simulink model "SecRwLtStBkReclnHolderChk"  (R2018b)
settings: Solver=FixedStepDiscrete  StartTime=0.0  StopTime=10.0  FixedStep=0.01  RelTol=1e-3
libraries: simulink x2
settings Model: Creator=sn2xws  LastModifiedBy=sn2xws
settings Model: ModifiedHistory=|
  | 2023/11/7
  | bug 555794 童锁需要停止21-26
  | 2024.5.8 V3.0.0 557 eze模式变更
  | 2024.9.9 V3.0.1 新增Md56
  | 25.7.7 V3.13.0 新增Md61 Md62
settings DataIOCC: SaveFormat=StructureWithTime
settings OptimizationCC: DefaultParameterBehavior=Inlined  EnhancedBackFolding=on  PassReuseOutputArgsAs=Individual arguments  ZeroExternalMemoryAtStartup=off  ZeroInternalMemoryAtStartup=off  OptimizeBlockOrder=speed  DifferentSizesBufferReuse=on  OptimizationCustomize=off
settings DebuggingCC: ParameterTunabilityLossMsg=error
settings ModelReferenceCC: ModelReferenceNumInstancesAllowed=Single
settings SFSimCC: MATLABDynamicMemAlloc=off
settings RTWCC: SystemTargetFile=autosar.tlc  GenCodeOnly=on  TemplateMakefile=ert_default_tmf  Description=AUTOSAR  GenerateReport=on  IncludeHyperlinkInReport=on  LaunchReport=on  GenerateTraceInfo=on  GenerateTraceReport=on  GenerateTraceReportSl=on  GenerateTraceReportSf=on  GenerateTraceReportEml=on  GenerateCodeMetricsReport=on
settings CodeAppCC: ForceParamTrailComments=on  IgnoreCustomStorageClasses=off  OperatorAnnotations=on  SimulinkDataObjDesc=on  SFDataObjDesc=on  InsertBlockDesc=on
settings STFCustomTargetCC: TargetLangStandard=C99 (ISO)  MultiwordLength=256  ParMdlRefBuildCompliant=on  CompOptLevelCompliant=on  IncludeMdlTerminateFcn=off  CombineOutputUpdateFcns=on  SuppressErrorStatus=on  ERTCustomFileBanners=on  SupportNonFinite=off  SupportComplex=off  SupportContinuousTime=off  SupportNonInlinedSFcns=off  RemoveResetFunc=on  MATLABClassNameForMDSCustomization=Simulink.SoftwareTarget.ERTCustomization  AutosarCompliant=on  UseToolchainInfoCompliant=on  LookupTableObjectStructAxisOrder=2,1,3,4,...  LUTObjectStructOrderEvenSpacing=Size,Table,Breakpoints  SystemTargetFile=autosar.tlc
settings ERTTargetCC: TargetLangStandard=C99 (ISO)  ConcurrentExecutionCompliant=off  IncludeMdlTerminateFcn=off  SuppressErrorStatus=on  SupportNonFinite=off  SupportComplex=off  ModelStepFunctionPrototypeControlCompliant=off  CPPClassGenCompliant=off  AutosarCompliant=on  LookupTableObjectStructAxisOrder=2,1,3,4,...  LUTObjectStructOrderEvenSpacing=Size,Table,Breakpoints  InlinedParameterPlacement=NonHierarchical  ERTCustomFileTemplate=example_file_process.tlc  ERTFilePackagingFormat=Compact

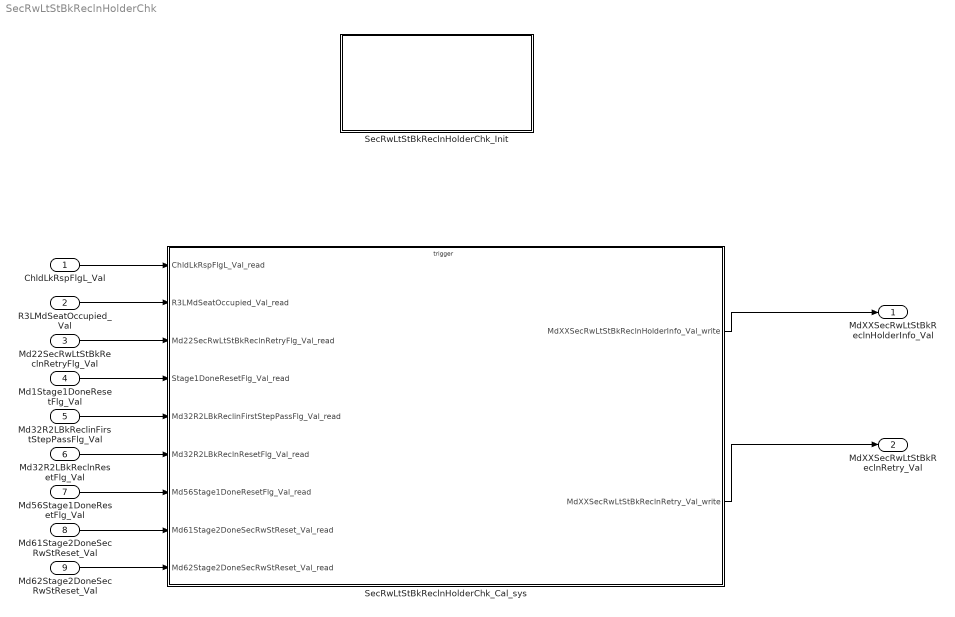
== system SecRwLtStBkReclnHolderChk ==
  ChldLkRspFlgL_Val : Inport  OutDataTypeStr=boolean  PortDimensions=1
  R3LMdSeatOccupied_Val : Inport  Port=2  OutDataTypeStr=boolean  PortDimensions=1
  Md22SecRwLtStBkReclnRetryFlg_Val : Inport  Port=3  OutDataTypeStr=boolean  PortDimensions=1
  Md1Stage1DoneResetFlg_Val : Inport  Port=4  OutDataTypeStr=boolean  PortDimensions=1
  Md32R2LBkReclinFirstStepPassFlg_Val : Inport  Port=5  OutDataTypeStr=boolean  PortDimensions=1
  Md32R2LBkReclnResetFlg_Val : Inport  Port=6  OutDataTypeStr=boolean  PortDimensions=1
  Md56Stage1DoneResetFlg_Val : Inport  Port=7  OutDataTypeStr=boolean  PortDimensions=1
  Md61Stage2DoneSecRwStReset_Val : Inport  Port=8  OutDataTypeStr=boolean  PortDimensions=1
  Md62Stage2DoneSecRwStReset_Val : Inport  Port=9  OutDataTypeStr=boolean  PortDimensions=1
  SecRwLtStBkReclnHolderChk_Cal_sys : Subsystem
  SecRwLtStBkReclnHolderChk_Init : Subsystem
  MdXXSecRwLtStBkReclnHolderInfo_Val : Outport  OutDataTypeStr=uint32  PortDimensions=1
  MdXXSecRwLtStBkReclnRetry_Val : Outport  Port=2  OutDataTypeStr=uint32  PortDimensions=1
  wires:
  ChldLkRspFlgL_Val/1 -> SecRwLtStBkReclnHolderChk_Cal_sys/1(ChldLkRspFlgL_Val_read)
  R3LMdSeatOccupied_Val/1 -> SecRwLtStBkReclnHolderChk_Cal_sys/2(R3LMdSeatOccupied_Val_read)
  SecRwLtStBkReclnHolderChk_Cal_sys/1(MdXXSecRwLtStBkReclnHolderInfo_Val_write) -> MdXXSecRwLtStBkReclnHolderInfo_Val/1
  Md22SecRwLtStBkReclnRetryFlg_Val/1 -> SecRwLtStBkReclnHolderChk_Cal_sys/3(Md22SecRwLtStBkReclnRetryFlg_Val_read)
  SecRwLtStBkReclnHolderChk_Cal_sys/2(MdXXSecRwLtStBkReclnRetry_Val_write) -> MdXXSecRwLtStBkReclnRetry_Val/1
  Md1Stage1DoneResetFlg_Val/1 -> SecRwLtStBkReclnHolderChk_Cal_sys/4(Stage1DoneResetFlg_Val_read)
  Md32R2LBkReclinFirstStepPassFlg_Val/1 -> SecRwLtStBkReclnHolderChk_Cal_sys/5(Md32R2LBkReclinFirstStepPassFlg_Val_read)
  Md32R2LBkReclnResetFlg_Val/1 -> SecRwLtStBkReclnHolderChk_Cal_sys/6(Md32R2LBkReclnResetFlg_Val_read)
  Md56Stage1DoneResetFlg_Val/1 -> SecRwLtStBkReclnHolderChk_Cal_sys/7(Md56Stage1DoneResetFlg_Val_read)
  Md61Stage2DoneSecRwStReset_Val/1 -> SecRwLtStBkReclnHolderChk_Cal_sys/8(Md61Stage2DoneSecRwStReset_Val_read)
  Md62Stage2DoneSecRwStReset_Val/1 -> SecRwLtStBkReclnHolderChk_Cal_sys/9(Md62Stage2DoneSecRwStReset_Val_read)

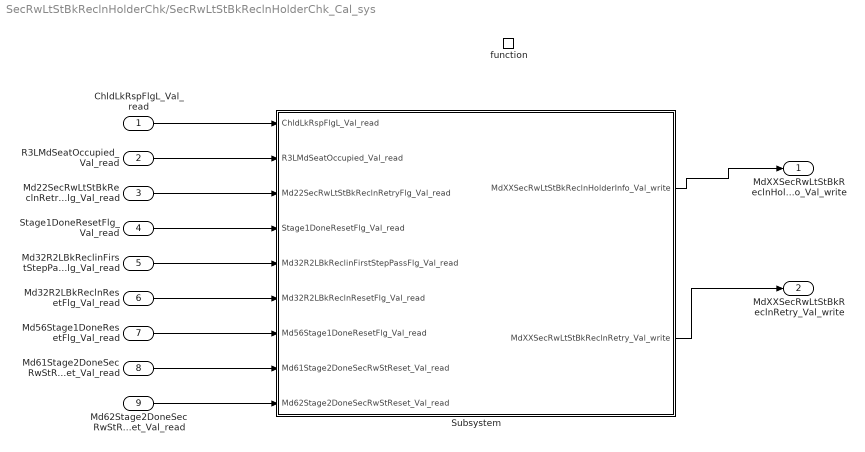
== system SecRwLtStBkReclnHolderChk/SecRwLtStBkReclnHolderChk_Cal_sys ==
  ChldLkRspFlgL_Val_read : Inport
  R3LMdSeatOccupied_Val_read : Inport  Port=2
  Md22SecRwLtStBkReclnRetryFlg_Val_read : Inport  Port=3
  Stage1DoneResetFlg_Val_read : Inport  Port=4
  Md32R2LBkReclinFirstStepPassFlg_Val_read : Inport  Port=5
  Md32R2LBkReclnResetFlg_Val_read : Inport  Port=6
  Md56Stage1DoneResetFlg_Val_read : Inport  Port=7
  Md61Stage2DoneSecRwStReset_Val_read : Inport  Port=8
  Md62Stage2DoneSecRwStReset_Val_read : Inport  Port=9
  function : TriggerPort  TriggerType=function-call  IsSimulinkFunction=on  FunctionName=SecRwLtStBkReclnHolderChk_Cal  VariantControl=(inherit)
  Subsystem : Subsystem
  MdXXSecRwLtStBkReclnHolderInfo_Val_write : Outport
      settings: EnsureOutportIsVirtual=on
  MdXXSecRwLtStBkReclnRetry_Val_write : Outport  Port=2
      settings: EnsureOutportIsVirtual=on
  wires:
  Subsystem/1(MdXXSecRwLtStBkReclnHolderInfo_Val_write) -> MdXXSecRwLtStBkReclnHolderInfo_Val_write/1
  ChldLkRspFlgL_Val_read/1 -> Subsystem/1(ChldLkRspFlgL_Val_read)
  R3LMdSeatOccupied_Val_read/1 -> Subsystem/2(R3LMdSeatOccupied_Val_read)
  Md22SecRwLtStBkReclnRetryFlg_Val_read/1 -> Subsystem/3(Md22SecRwLtStBkReclnRetryFlg_Val_read)
  Subsystem/2(MdXXSecRwLtStBkReclnRetry_Val_write) -> MdXXSecRwLtStBkReclnRetry_Val_write/1
  Stage1DoneResetFlg_Val_read/1 -> Subsystem/4(Stage1DoneResetFlg_Val_read)
  Md32R2LBkReclnResetFlg_Val_read/1 -> Subsystem/6(Md32R2LBkReclnResetFlg_Val_read)
  Md32R2LBkReclinFirstStepPassFlg_Val_read/1 -> Subsystem/5(Md32R2LBkReclinFirstStepPassFlg_Val_read)
  Md56Stage1DoneResetFlg_Val_read/1 -> Subsystem/7(Md56Stage1DoneResetFlg_Val_read)
  Md61Stage2DoneSecRwStReset_Val_read/1 -> Subsystem/8(Md61Stage2DoneSecRwStReset_Val_read)
  Md62Stage2DoneSecRwStReset_Val_read/1 -> Subsystem/9(Md62Stage2DoneSecRwStReset_Val_read)

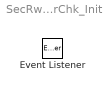
== system SecRwLtStBkReclnHolderChk/SecRwLtStBkReclnHolderChk_Init ==
  Event Listener : EventListener  EventName=reset

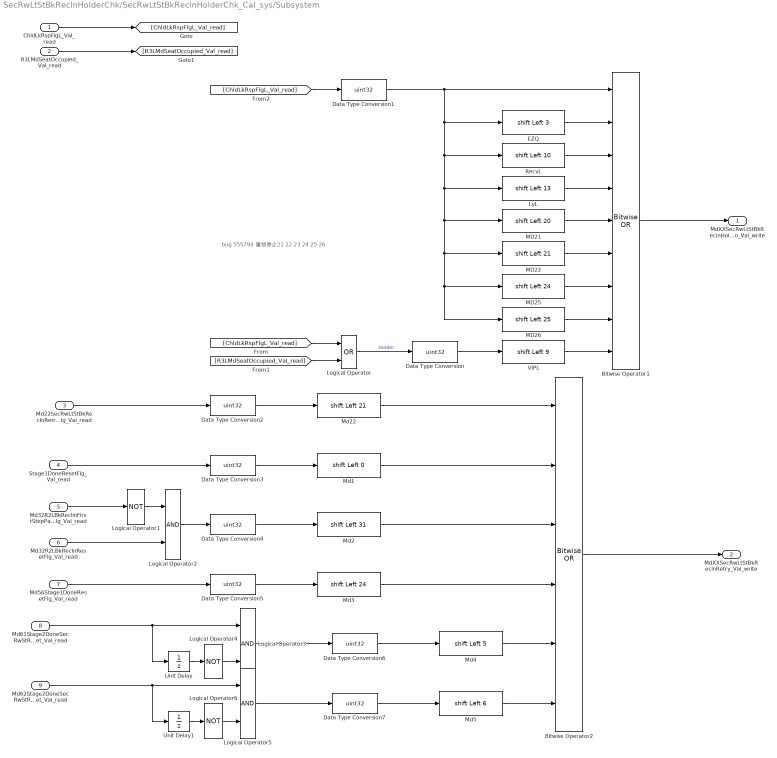
== system SecRwLtStBkReclnHolderChk/SecRwLtStBkReclnHolderChk_Cal_sys/Subsystem ==
  note: bug 555794 童锁停止21 22 23 24 25 26
  ChldLkRspFlgL_Val_read : Inport
  R3LMdSeatOccupied_Val_read : Inport  Port=2
  Md22SecRwLtStBkReclnRetryFlg_Val_read : Inport  Port=3
  Stage1DoneResetFlg_Val_read : Inport  Port=4
  Md32R2LBkReclinFirstStepPassFlg_Val_read : Inport  Port=5
  Md32R2LBkReclnResetFlg_Val_read : Inport  Port=6
  Md56Stage1DoneResetFlg_Val_read : Inport  Port=7
  Md61Stage2DoneSecRwStReset_Val_read : Inport  Port=8
  Md62Stage2DoneSecRwStReset_Val_read : Inport  Port=9
  Bitwise Operator1 : simulink/Logic and Bit Operations/Bitwise Operator  logicop=OR  UseBitMask=off  NumInputPorts=9  BitMask=bin2dec('11011001')  BitMaskRealWorld=Stored Integer
  Bitwise Operator2 : simulink/Logic and Bit Operations/Bitwise Operator  logicop=OR  UseBitMask=off  NumInputPorts=6  BitMask=bin2dec('11011001')  BitMaskRealWorld=Stored Integer
  Data Type Conversion{,1..7} (8 alike) : DataTypeConversion  OutDataTypeStr=uint32
  EZQ : ArithShift  BitShiftNumber=3  BitShiftDirection=Left
  Logical Operator : Logic  Operator=OR  AllPortsSameDT=off  OutDataTypeStr=boolean
  Logical Operator1 : Logic  Operator=NOT  AllPortsSameDT=off  OutDataTypeStr=boolean
  Logical Operator2 : Logic  AllPortsSameDT=off  OutDataTypeStr=boolean
  Logical Operator3 : Logic  AllPortsSameDT=off  OutDataTypeStr=boolean
  Logical Operator4 : Logic  Operator=NOT  AllPortsSameDT=off  OutDataTypeStr=boolean
  Logical Operator5 : Logic  AllPortsSameDT=off  OutDataTypeStr=boolean
  Logical Operator6 : Logic  Operator=NOT  AllPortsSameDT=off  OutDataTypeStr=boolean
  LyL : ArithShift  BitShiftNumber=13  BitShiftDirection=Left
  MD21 : ArithShift  BitShiftNumber=20  BitShiftDirection=Left
  MD22 : ArithShift  BitShiftNumber=21  BitShiftDirection=Left
  MD25 : ArithShift  BitShiftNumber=24  BitShiftDirection=Left
  MD26 : ArithShift  BitShiftNumber=25  BitShiftDirection=Left
  Md1 : ArithShift  BitShiftDirection=Left
  Md2 : ArithShift  BitShiftNumber=31  BitShiftDirection=Left
  Md22 : ArithShift  BitShiftNumber=21  BitShiftDirection=Left
  Md3 : ArithShift  BitShiftNumber=24  BitShiftDirection=Left
  Md4 : ArithShift  BitShiftNumber=5  BitShiftDirection=Left
  Md5 : ArithShift  BitShiftNumber=6  BitShiftDirection=Left
  RecvL : ArithShift  BitShiftNumber=10  BitShiftDirection=Left
  Unit Delay : UnitDelay  SampleTime=-1
  Unit Delay1 : UnitDelay  SampleTime=-1
  VIPL : ArithShift  BitShiftNumber=9  BitShiftDirection=Left
  MdXXSecRwLtStBkReclnHolderInfo_Val_write : Outport
      settings: EnsureOutportIsVirtual=on
  MdXXSecRwLtStBkReclnRetry_Val_write : Outport  Port=2
      settings: EnsureOutportIsVirtual=on
  wires:
  R3LMdSeatOccupied_Val_read/1 -> [R3LMdSeatOccupied_Val_read]
  ChldLkRspFlgL_Val_read/1 -> [ChldLkRspFlgL_Val_read]
  Bitwise Operator1/1 -> MdXXSecRwLtStBkReclnHolderInfo_Val_write/1
  [R3LMdSeatOccupied_Val_read] -> Logical Operator/2
  [ChldLkRspFlgL_Val_read] -> Logical Operator/1
  Data Type Conversion/1 -> VIPL/1
  Logical Operator/1 -> Data Type Conversion/1  "Holder"
  [ChldLkRspFlgL_Val_read] -> Data Type Conversion1/1
  EZQ/1 -> Bitwise Operator1/2
  RecvL/1 -> Bitwise Operator1/3
  LyL/1 -> Bitwise Operator1/4
  VIPL/1 -> Bitwise Operator1/9
  Md22SecRwLtStBkReclnRetryFlg_Val_read/1 -> Data Type Conversion2/1
  Data Type Conversion2/1 -> Md22/1
  MD21/1 -> Bitwise Operator1/5
  MD22/1 -> Bitwise Operator1/6
  MD25/1 -> Bitwise Operator1/7
  MD26/1 -> Bitwise Operator1/8
  Data Type Conversion1/1 -> MD26/1, MD25/1, MD22/1, MD21/1, LyL/1, RecvL/1, EZQ/1, Bitwise Operator1/1
  Stage1DoneResetFlg_Val_read/1 -> Data Type Conversion3/1
  Data Type Conversion3/1 -> Md1/1
  Bitwise Operator2/1 -> MdXXSecRwLtStBkReclnRetry_Val_write/1
  Md22/1 -> Bitwise Operator2/1
  Md1/1 -> Bitwise Operator2/2
  Md32R2LBkReclnResetFlg_Val_read/1 -> Logical Operator2/2
  Md32R2LBkReclinFirstStepPassFlg_Val_read/1 -> Logical Operator1/1
  Logical Operator1/1 -> Logical Operator2/1
  Logical Operator2/1 -> Data Type Conversion4/1
  Data Type Conversion4/1 -> Md2/1
  Md2/1 -> Bitwise Operator2/3
  Data Type Conversion5/1 -> Md3/1
  Md56Stage1DoneResetFlg_Val_read/1 -> Data Type Conversion5/1
  Md3/1 -> Bitwise Operator2/4
  Md4/1 -> Bitwise Operator2/5
  Data Type Conversion6/1 -> Md4/1
  Logical Operator3/1 -> Data Type Conversion6/1
  Md61Stage2DoneSecRwStReset_Val_read/1 -> Logical Operator3/1, Unit Delay/1
  Unit Delay/1 -> Logical Operator4/1
  Logical Operator4/1 -> Logical Operator3/2
  Logical Operator6/1 -> Logical Operator5/2
  Unit Delay1/1 -> Logical Operator6/1
  Md62Stage2DoneSecRwStReset_Val_read/1 -> Logical Operator5/1, Unit Delay1/1
  Logical Operator5/1 -> Data Type Conversion7/1
  Data Type Conversion7/1 -> Md5/1
  Md5/1 -> Bitwise Operator2/6
